simulink model "PubIfDecisionLM_MDL"  (R2020b)
settings: configuration reference "DspaceConfig" (kept outside this file)
PostLoadFcn:
  | if any(exist('dsrtsu_mdlpostloadfcn', 'file') ~= 0), dsrtsu_mdlpostloadfcn('Execute', bdroot); end
InitFcn:
  | , if any(exist('dsmpb_private', 'file') ~= 0), dsmpb_private('dsmpb_mdlclblib', 'Init', bdroot); end,
undefined symbols (not defined in the file or in its folder): OFM_OBJ_FUSIONTYPE_E, OFM_OBJ_MOVINGSTATE_E, OFM_OBJ_ORIENTATION_E, OFM_OBJ_TYPE_E, P_LM_Cyc, P_LM_EMLHistKapRcdBufSize, P_LM_EMLHistTrajBaseDis, P_LM_EMLHistTrajPNum, P_LM_EMLKapCorrMaxThre, P_LM_EMLMinKapThre, P_LM_EMLPathDisDiffThre, P_LM_EMLQuaFiltPar, P_LM_EMLTurnActKapThre, P_LM_EMLValidQuaThre, P_LM_FntPath1Disgap, P_LM_FntPath1MinDis, P_LM_FntPath1Timegap, P_LM_FntPath2Disgap, P_LM_FntPath2MinDis, P_LM_FntPath2Timegap, P_LM_FntPath3Disgap, P_LM_FntPath3MinDis, P_LM_FntPath3Timegap, P_LM_FusBLParFiltP, P_LM_FusEVDifC2Thre, P_LM_FusEVOPath1AllVSLDisThre, P_LM_FusEVOPath1AllVSLLostNumThre, P_LM_FusEVOPath1AllVSLQuaThre, P_LM_FusEVOPath1OTLFacNLC, P_LM_FusOTLQuaThre, P_LM_FusOTLSW, P_LM_FusParC0Index, P_LM_FusParC1Index, P_LM_FusParC2Index, P_LM_FusParC3Index, P_LM_FusVSLQuaThre, P_LM_FusVSLSW, P_LM_FusVSLValidSteerWheerAngThre, P_LM_FusVSLValidVxvThre, P_LM_LaneWidth, P_LM_OTLBufTPInfoEvaFactor, P_LM_OTLObjNum, P_LM_OTLObjSelectAgeThre, P_LM_OTLObjSelectDxAssessVx, P_LM_OTLObjSelectDxThre, P_LM_OTLObjSelectVxThre, P_LM_OTLObjSelectVyAssessDx, P_LM_OTLObjSelectVyThre, P_LM_OTLTrajPntBaseDis, P_LM_OTLTrajStdThre, P_LM_VSLAvailLineNum, P_LM_VSLBLSDiffThre, P_LM_VSLBLSDisRatio, P_LM_VSLFusBLParFiltP_C1, P_LM_VSLFusBLParFiltP_C2, P_LM_VSLFusBLParFiltP_C3, P_LM_VSLFusBLParFiltP_Quality, P_LM_VSLHistTrajBaseDis, P_LM_VSLHistTrajPNum, P_LM_VSLLCC0diff ... (+18)
libraries: simulink x145, LM_LIB x43
(part 3 of 24)

== system PubIfDecisionLM_MDL/Subsystem2/LM_EML/LM_EMLFntPath1/LM_EML_C0 ==
  LM_DrivInWLType : Inport
  Constant : Constant  Value=P_LM_LaneWidth  OutDataTypeStr=single
  Merge{,1..3} (4 alike) : Merge  Inputs=3
  Switch Case : SwitchCase  CaseConditions={[0,2],1,3}  ShowDefaultCase=off
  Switch Case Action Subsystem : Subsystem  TreatAsAtomicUnit=on
  Switch Case Action Subsystem1 : Subsystem  TreatAsAtomicUnit=on
  Switch Case Action Subsystem2 : Subsystem  TreatAsAtomicUnit=on
  LM_EMLLLC0 : Outport
  LM_EMLLRC0 : Outport  Port=2
  LM_EMLRLC0 : Outport  Port=3
  LM_EMLRRC0 : Outport  Port=4
  wires:
  Merge3/1 -> LM_EMLRRC0/1  "LM_EMLRRC0"
  Merge2/1 -> LM_EMLRLC0/1  "LM_EMLRLC0"
  Merge1/1 -> LM_EMLLRC0/1  "LM_EMLLRC0"
  Switch Case Action Subsystem2/4(LM_EML_RRC0) -> Merge3/3
  Switch Case Action Subsystem1/4(LM_EML_RRC0) -> Merge3/2
  Switch Case Action Subsystem/4(LM_EML_RRC0) -> Merge3/1
  Switch Case Action Subsystem2/3(LM_EML_RLC0) -> Merge2/3
  Switch Case Action Subsystem1/3(LM_EML_RLC0) -> Merge2/2
  Switch Case Action Subsystem1/2(LM_EML_LRC0) -> Merge1/2
  Switch Case Action Subsystem1/1(LM_EML_LLC0) -> Merge/2
  Switch Case Action Subsystem/3(LM_EML_RLC0) -> Merge2/1
  Switch Case Action Subsystem2/2(LM_EML_LRC0) -> Merge1/3
  Switch Case Action Subsystem/2(LM_EML_LRC0) -> Merge1/1
  Switch Case Action Subsystem2/1(LM_EML_LLC0) -> Merge/3
  Merge/1 -> LM_EMLLLC0/1  "LM_EMLLLC0"
  Switch Case Action Subsystem/1(LM_EML_LLC0) -> Merge/1
  Constant/1 -> Switch Case Action Subsystem/1(P_LM_LaneWidth), Switch Case Action Subsystem1/1(P_LM_LaneWidth), Switch Case Action Subsystem2/1(P_LM_LaneWidth)
  Switch Case/3 -> Switch Case Action Subsystem2/Action
  Switch Case/2 -> Switch Case Action Subsystem1/Action
  Switch Case/1 -> Switch Case Action Subsystem/Action
  LM_DrivInWLType/1 -> Switch Case/1

== system PubIfDecisionLM_MDL/Subsystem2/LM_EML/LM_EMLRearPath1/LM_EMLEgoTrajRecorddFlgCalc ==
  note: 0x0: not standstill
  VehStandstill : Inport
  VxvRef_ms : Inport  Port=2
  Add : Sum
  Compare To Zero : simulink/Logic and Bit Operations/Compare To Zero  relop===  OutDataTypeStr=boolean
  Constant : Constant  Value=0  OutDataTypeStr=boolean
  Constant1 : Constant  OutDataTypeStr=uint8
  Constant2 : Constant  Value=0
  Constant3 : Constant  Value=0.0001  OutDataTypeStr=single
  Constant4 : Constant  Value=P_LM_EMLHistTrajBaseDis  OutDataTypeStr=single
  Constant6 : Constant  Value=P_LM_Cyc
  Data Type Conversion : DataTypeConversion  OutDataTypeStr=uint8
  Divide : Product  Inputs=*/
  Divide1 : Product  Inputs=*/
  Relational Operator : RelationalOperator  Operator=<=  OutDataTypeStr=boolean  RndMeth=Nearest
  Switch : Switch  Criteria=u2 ~= 0
  Switch1 : Switch  Criteria=u2 ~= 0
  Switch2 : Switch  Criteria=u2 ~= 0
  Unit Delay : UnitDelay  SampleTime=-1  HasFrameUpgradeWarning=on
  LM_EMLHistTrajRcdFlg : Outport
  wires:
  Constant4/1 -> Divide/1
  Switch2/1 -> Divide/2
  Divide/1 -> Divide1/1
  Constant6/1 -> Divide1/2
  Constant/1 -> Switch/1
  Switch/1 -> LM_EMLHistTrajRcdFlg/1  "LM_EMLHistTrajRcdFlg"
  Unit Delay/1 -> Add/2
  Constant1/1 -> Add/1
  Divide1/1 -> Data Type Conversion/1
  Add/1 -> Relational Operator/2, Switch1/3
  Constant2/1 -> Switch1/1
  Switch1/1 -> Unit Delay/1
  Data Type Conversion/1 -> Relational Operator/1
  Relational Operator/1 -> Switch/3, Switch1/2
  VehStandstill/1 -> Switch/2
  VxvRef_ms/1 -> Switch2/3, Compare To Zero/1
  Compare To Zero/1 -> Switch2/2
  Constant3/1 -> Switch2/1

== system PubIfDecisionLM_MDL/Subsystem2/LM_EML/LM_EMLRearPath1/LM_EMLHistTrajCoordinateConvert ==
  note: 0x0: not standstill
  LM_EMLHistTrajVectXK1 : Inport
  LM_EMLHistTrajVectYK1 : Inport  Port=2
  LM_ComEVOffsetX : Inport  Port=3
  LM_ComEVOffsetY : Inport  Port=4
  LM_ComEVOffsetAng : Inport  Port=5
  VehStandstill : Inport  Port=6
  If : If  IfExpression=u1 == 0
  If Action Subsystem : Subsystem  TreatAsAtomicUnit=on
  If Action Subsystem1 : Subsystem  TreatAsAtomicUnit=on
  Merge : Merge
  Merge1 : Merge
  LM_EMLHistTrajVectXK1Adju : Outport
  LM_EMLHistTrajVectYK1Adju : Outport  Port=2
  wires:
  Merge1/1 -> LM_EMLHistTrajVectYK1Adju/1
  Merge/1 -> LM_EMLHistTrajVectXK1Adju/1
  If Action Subsystem1/2(LM_EMLHistTrajVectYK1Adju) -> Merge1/2
  If Action Subsystem/2(LM_EMLHistTrajVectYK1Adju) -> Merge1/1
  If Action Subsystem1/1(LM_EMLHistTrajVectXK1Adju) -> Merge/2
  If Action Subsystem/1(LM_EMLHistTrajVectXK1Adju) -> Merge/1
  LM_ComEVOffsetX/1 -> If Action Subsystem/1(LM_ComEVOffsetX)
  LM_ComEVOffsetY/1 -> If Action Subsystem/2(LM_ComEVOffsetY)
  LM_ComEVOffsetAng/1 -> If Action Subsystem/3(LM_ComEVOffsetAng)
  LM_EMLHistTrajVectXK1/1 -> If Action Subsystem/4(LM_EMLHistTrajVectXK1), If Action Subsystem1/1(LM_EMLHistTrajVectXK1)
  LM_EMLHistTrajVectYK1/1 -> If Action Subsystem/5(LM_EMLHistTrajVectYK1), If Action Subsystem1/2(LM_EMLHistTrajVectYK1)
  If/2 -> If Action Subsystem1/Action
  If/1 -> If Action Subsystem/Action
  VehStandstill/1 -> If/1

== system PubIfDecisionLM_MDL/Subsystem2/LM_EML/LM_EMLRearPath1/LM_EMLHistTrajRecordBufferInfo ==
  LM_EMLHistTrajRcdFlg : Inport
  Add : Sum
  Add1 : Sum
  Add2 : Sum
  Compare To Zero{,1..3} (4 alike) : simulink/Logic and Bit Operations/Compare To Zero  relop===  OutDataTypeStr=boolean
  Constant{,2..4,7..9} (7 alike) : Constant  OutDataTypeStr=uint8
  Constant1 : Constant  Value=P_LM_EMLHistTrajPNum  OutDataTypeStr=uint8
  Constant5 : Constant  Value=P_LM_EMLHistTrajPNum  OutDataTypeStr=uint8
  Constant6 : Constant  Value=3  OutDataTypeStr=uint8
  Mod1 : Math  Operator=mod  SignedPower=on  SaturateOnIntegerOverflow=on
  Product : Product
  Relational Operator : RelationalOperator  Operator=>  OutDataTypeStr=boolean  RndMeth=Nearest
  Relational Operator1 : RelationalOperator  Operator=<=  OutDataTypeStr=boolean  RndMeth=Nearest
  Switch{,1..7} (8 alike) : Switch  Criteria=u2 ~= 0
  Unit Delay : UnitDelay  SampleTime=-1  HasFrameUpgradeWarning=on
  LM_EMLHistPEndPos : Outport
  LM_EMLHistPFristPos : Outport  Port=2
  LM_EMLHistPNum : Outport  Port=3
  wires:
  Switch2/1 -> Switch5/3  "LM_EMLHistPEndPos"
  Compare To Zero/1 -> Switch2/2
  Switch6/1 -> LM_EMLHistPEndPos/1  "LM_EMLHistPEndPos"
  LM_EMLHistTrajRcdFlg/1 -> Switch1/2
  Switch/1 -> LM_EMLHistPFristPos/1  "LM_EMLHistPFristPos"
  Constant3/1 -> Add2/2
  Mod1/1 -> Add1/1, Compare To Zero/1, Switch2/3
  Add2/1 -> Switch4/1
  Add1/1 -> Switch3/3
  Add/1 -> Switch1/1
  Switch1/1 -> Relational Operator1/1, Mod1/1, Switch4/3, Relational Operator/1, Switch5/1
  Relational Operator1/1 -> Switch3/2, Switch5/2
  Constant5/1 -> Product/1
  Product/1 -> Relational Operator/2
  Constant4/1 -> Add1/2
  Relational Operator/1 -> Switch4/2
  Constant1/1 -> Relational Operator1/2, Mod1/2, Add2/1, Switch2/1
  Constant2/1 -> Switch3/1
  Unit Delay/1 -> Switch1/3, Add/1
  Constant6/1 -> Product/2
  Constant/1 -> Add/2
  Switch3/1 -> Switch/3, Compare To Zero1/1
  Compare To Zero1/1 -> Switch/2
  Constant7/1 -> Switch/1
  Constant8/1 -> Switch6/1
  Compare To Zero2/1 -> Switch6/2
  Switch5/1 -> Compare To Zero2/1, Switch6/3
  Switch4/1 -> Switch7/3, Unit Delay/1, Compare To Zero3/1
  Compare To Zero3/1 -> Switch7/2
  Constant9/1 -> Switch7/1
  Switch7/1 -> LM_EMLHistPNum/1  "LM_EMLHistPNum"

== system PubIfDecisionLM_MDL/Subsystem2/LM_EML/LM_EMLRearPath1/LM_EMLHistTrajRecordBufferUpdate ==
  LM_EMLHistTrajVectXK1Adju : Inport
  LM_EMLHistTrajVectYK1Adju : Inport  Port=2
  LM_EMLHistTrajRcdFlg : Inport  Port=3
  LM_EMLHistPEndPos : Inport  Port=4
  Data Type Conversion : DataTypeConversion  OutDataTypeStr=single
  Data Type Conversion1 : DataTypeConversion  OutDataTypeStr=single
  MATLAB Function : MATLAB Function  TreatAsAtomicUnit=on
  MATLAB Function1 : MATLAB Function  TreatAsAtomicUnit=on
  Switch : Switch  Criteria=u2 ~= 0
  Switch2 : Switch  Criteria=u2 ~= 0
  LM_EMLHistTrajVectX : Outport
  LM_EMLHistTrajVectY : Outport  Port=2
  wires:
  MATLAB Function1/1(LM_EMLHistTrajVectX) -> Switch2/1
  MATLAB Function/1(LM_EMLHistTrajVectX) -> Switch/1
  LM_EMLHistPEndPos/1 -> MATLAB Function/1(LM_EMLHistPEndPos), MATLAB Function1/1(LM_EMLHistPEndPos)
  LM_EMLHistTrajVectXK1Adju/1 -> MATLAB Function/2(LM_EMLHistTrajVectXK1Adju), Switch/3
  LM_EMLHistTrajRcdFlg/1 -> Switch2/2, Switch/2
  LM_EMLHistTrajVectYK1Adju/1 -> Switch2/3, MATLAB Function1/2(LM_EMLHistTrajVectXK1Adju)
  Switch2/1 -> Data Type Conversion1/1
  Switch/1 -> Data Type Conversion/1
  Data Type Conversion/1 -> LM_EMLHistTrajVectX/1
  Data Type Conversion1/1 -> LM_EMLHistTrajVectY/1

== system PubIfDecisionLM_MDL/Subsystem2/LM_Fusion1/LM_FusBaseLineFilt/LM_FusBaseLineC0Filt ==
  note: P_LM_FusBLParFiltP
  note: P_LM_FusBLParFiltP
  note: P_LM_FusBLParFiltP
  note: P_LM_FusBLParFiltP
  DIR_LC2LeValid : Inport
  DIR_LC2RigValid : Inport  Port=2
  LM_LLC0BefFilt : Inport  Port=3
  LM_LRC0BefFilt : Inport  Port=4
  LM_RLC0BefFilt : Inport  Port=5
  LM_RRC0BefFilt : Inport  Port=6
  Add{1..3,12} (4 alike) : Sum
  Compare To Zero{,1..3} (4 alike) : simulink/Logic and Bit Operations/Compare To Zero  relop===  OutDataTypeStr=boolean
  Constant{1..3,10} (4 alike) : Constant  Value=P_LM_FusBLParFiltP  OutDataTypeStr=single
  Logical Operator : Logic  Operator=OR  AllPortsSameDT=off  OutDataTypeStr=boolean
  Product{1..3,17} (4 alike) : Product
  Subtract{1..4} (4 alike) : Sum  Inputs=+-
  Switch{,1..7} (8 alike) : Switch  Criteria=u2 ~= 0
  Unit Delay{1..4} (4 alike) : UnitDelay  SampleTime=-1  HasFrameUpgradeWarning=on
  LM_LLC0 : Outport
  LM_LRC0 : Outport  Port=2
  LM_RLC0 : Outport  Port=3
  LM_RRC0 : Outport  Port=4
  wires:
  Constant10/1 -> Product17/2
  Add12/1 -> Switch4/3
  Unit Delay2/1 -> Compare To Zero/1, Add12/2, Subtract2/2
  Subtract2/1 -> Product17/1
  Product17/1 -> Add12/1
  LM_LLC0BefFilt/1 -> Subtract2/1, Switch4/1, Switch/1
  DIR_LC2LeValid/1 -> Logical Operator/1
  DIR_LC2RigValid/1 -> Logical Operator/2
  Logical Operator/1 -> Switch3/2, Switch2/2, Switch1/2, Switch/2
  Constant1/1 -> Product1/2
  Add1/1 -> Switch5/3
  Unit Delay1/1 -> Compare To Zero1/1, Add1/2, Subtract1/2
  Subtract1/1 -> Product1/1
  Product1/1 -> Add1/1
  LM_LRC0BefFilt/1 -> Switch5/1, Switch1/1, Subtract1/1
  Product2/1 -> Add2/1
  Subtract3/1 -> Product2/1
  Unit Delay3/1 -> Compare To Zero2/1, Add2/2, Subtract3/2
  Constant2/1 -> Product2/2
  LM_RLC0BefFilt/1 -> Switch6/1, Switch2/1, Subtract3/1
  Product3/1 -> Add3/1
  Subtract4/1 -> Product3/1
  Unit Delay4/1 -> Compare To Zero3/1, Add3/2, Subtract4/2
  Constant3/1 -> Product3/2
  Switch/1 -> LM_LLC0/1, Unit Delay2/1  "LM_LLC0"
  Switch1/1 -> LM_LRC0/1, Unit Delay1/1  "LM_LRC0"
  Switch2/1 -> LM_RLC0/1, Unit Delay3/1  "LM_RLC0"
  Switch3/1 -> LM_RRC0/1, Unit Delay4/1  "LM_RRC0"
  Switch4/1 -> Switch/3  "LM_LLC0"
  Compare To Zero/1 -> Switch4/2
  Compare To Zero1/1 -> Switch5/2
  Switch5/1 -> Switch1/3  "LM_LLC0"
  Switch6/1 -> Switch2/3  "LM_LLC0"
  Add2/1 -> Switch6/3
  Compare To Zero2/1 -> Switch6/2
  Compare To Zero3/1 -> Switch7/2
  Add3/1 -> Switch7/3
  LM_RRC0BefFilt/1 -> Subtract4/1, Switch3/1, Switch7/1
  Switch7/1 -> Switch3/3  "LM_LLC0"

== system PubIfDecisionLM_MDL/Subsystem2/LM_Fusion1/LM_FusBaseLineFilt/LM_FusBaseLineInfoFilt ==
  LM_FusBLInfo : Inport
  Bus Creator{,1..5} (6 alike) : BusCreator  Inputs=5  OutDataTypeStr=Bus: LM_FusBLPathInfoBus
  Bus Selector : BusSelector  OutputSignals=LM_FusBLFntPath1Info.LM_FusBLPathC0,LM_FusBLFntPath1Info.LM_FusBLPathC1,LM_FusBLFntPath1Info.LM_FusBLPathC2,LM_FusBLFntPath1Info.LM_FusBLPathC3,LM_FusBLFntPath1Info.LM_FusBLPathQuality
  Bus Selector1 : BusSelector  OutputSignals=LM_FusBLFntPath2Info.LM_FusBLPathC0,LM_FusBLFntPath2Info.LM_FusBLPathC1,LM_FusBLFntPath2Info.LM_FusBLPathC2,LM_FusBLFntPath2Info.LM_FusBLPathC3,LM_FusBLFntPath2Info.LM_FusBLPathQuality
  Bus Selector2 : BusSelector  OutputSignals=LM_FusBLFntPath3Info.LM_FusBLPathC0,LM_FusBLFntPath3Info.LM_FusBLPathC1,LM_FusBLFntPath3Info.LM_FusBLPathC2,LM_FusBLFntPath3Info.LM_FusBLPathC3,LM_FusBLFntPath3Info.LM_FusBLPathQuality
  Bus Selector3 : BusSelector  OutputSignals=LM_FusBLRearPath1Info.LM_FusBLPathC0,LM_FusBLRearPath1Info.LM_FusBLPathC1,LM_FusBLRearPath1Info.LM_FusBLPathC2,LM_FusBLRearPath1Info.LM_FusBLPathC3,LM_FusBLRearPath1Info.LM_FusBLPathQuality
  Bus Selector4 : BusSelector  OutputSignals=LM_FusBLRearPath2Info.LM_FusBLPathC0,LM_FusBLRearPath2Info.LM_FusBLPathC1,LM_FusBLRearPath2Info.LM_FusBLPathC2,LM_FusBLRearPath2Info.LM_FusBLPathC3,LM_FusBLRearPath2Info.LM_FusBLPathQuality
  Bus Selector5 : BusSelector  OutputSignals=LM_FusBLRearPath3Info.LM_FusBLPathC0,LM_FusBLRearPath3Info.LM_FusBLPathC1,LM_FusBLRearPath3Info.LM_FusBLPathC2,LM_FusBLRearPath3Info.LM_FusBLPathC3,LM_FusBLRearPath3Info.LM_FusBLPathQuality
  LM_FusBLFntPath1InfoFilt : Subsystem
  LM_FusBLFntPath2InfoFilt : LM_LIB/LM_FusBLPathInfoFilt  SystemSampleTime=-1  VariantActivationTime=update diagram  Latency=0  AutoFrameSizeCalculation=off
  LM_FusBLFntPath3InfoFilt : LM_LIB/LM_FusBLPathInfoFilt  SystemSampleTime=-1  VariantActivationTime=update diagram  Latency=0  AutoFrameSizeCalculation=off
  LM_FusBLRearPath1InfoFilt : LM_LIB/LM_FusBLPathInfoFilt  SystemSampleTime=-1  VariantActivationTime=update diagram  Latency=0  AutoFrameSizeCalculation=off
  LM_FusBLRearPath2InfoFilt : LM_LIB/LM_FusBLPathInfoFilt  SystemSampleTime=-1  VariantActivationTime=update diagram  Latency=0  AutoFrameSizeCalculation=off
  LM_FusBLRearPath3InfoFilt : LM_LIB/LM_FusBLPathInfoFilt  SystemSampleTime=-1  VariantActivationTime=update diagram  Latency=0  AutoFrameSizeCalculation=off
  Signal Conversion{,1..29} (30 alike) : SignalConversion  OverrideOpt=off
  LM_FusBLFntPath1Info : Outport
  LM_FusBLFntPath2Info : Outport  Port=2
  LM_FusBLFntPath3Info : Outport  Port=3
  LM_FusBLRearPath1Info : Outport  Port=4
  LM_FusBLRearPath2Info : Outport  Port=5
  LM_FusBLRearPath3Info : Outport  Port=6
  wires:
  Bus Selector/1 -> LM_FusBLFntPath1InfoFilt/1(LM_FusBLPathC0)  "<LM_FusBLPathC0>"
  Bus Selector/2 -> LM_FusBLFntPath1InfoFilt/2(LM_FusBLPathC1)  "<LM_FusBLPathC1>"
  Bus Selector/3 -> LM_FusBLFntPath1InfoFilt/3(LM_FusBLPathC2)  "<LM_FusBLPathC2>"
  Bus Selector/4 -> LM_FusBLFntPath1InfoFilt/4(LM_FusBLPathC3)  "<LM_FusBLPathC3>"
  Bus Selector/5 -> LM_FusBLFntPath1InfoFilt/5(LM_FusBLPathQuality)  "<LM_FusBLPathQuality>"
  Bus Creator/1 -> LM_FusBLFntPath1Info/1  "LM_FusBLFntPath1Info"
  LM_FusBLFntPath1InfoFilt/1(LM_FusBLPathC0Filt) -> Signal Conversion/1
  LM_FusBLFntPath1InfoFilt/2(LM_FusBLPathC1Filt) -> Signal Conversion1/1
  LM_FusBLFntPath1InfoFilt/3(LM_FusBLPathC2Filt) -> Signal Conversion2/1
  LM_FusBLFntPath1InfoFilt/4(LM_FusBLPathC3Filt) -> Signal Conversion3/1
  LM_FusBLFntPath1InfoFilt/5(LM_FusBLPathQualityFilt) -> Signal Conversion4/1
  LM_FusBLFntPath2InfoFilt/5 -> Signal Conversion9/1
  LM_FusBLFntPath2InfoFilt/4 -> Signal Conversion8/1
  LM_FusBLFntPath2InfoFilt/3 -> Signal Conversion7/1
  LM_FusBLFntPath2InfoFilt/2 -> Signal Conversion6/1
  LM_FusBLFntPath2InfoFilt/1 -> Signal Conversion5/1
  Bus Creator1/1 -> LM_FusBLFntPath2Info/1  "LM_FusBLFntPath2Info"
  Bus Creator2/1 -> LM_FusBLFntPath3Info/1  "LM_FusBLFntPath3Info"
  LM_FusBLFntPath3InfoFilt/1 -> Signal Conversion10/1
  LM_FusBLFntPath3InfoFilt/2 -> Signal Conversion11/1
  LM_FusBLFntPath3InfoFilt/3 -> Signal Conversion12/1
  LM_FusBLFntPath3InfoFilt/4 -> Signal Conversion13/1
  LM_FusBLFntPath3InfoFilt/5 -> Signal Conversion14/1
  LM_FusBLRearPath1InfoFilt/5 -> Signal Conversion24/1
  LM_FusBLRearPath1InfoFilt/4 -> Signal Conversion23/1
  LM_FusBLRearPath1InfoFilt/3 -> Signal Conversion22/1
  LM_FusBLRearPath1InfoFilt/2 -> Signal Conversion16/1
  LM_FusBLRearPath1InfoFilt/1 -> Signal Conversion15/1
  Bus Creator3/1 -> LM_FusBLRearPath1Info/1  "LM_FusBLRearPath1Info"
  Bus Creator4/1 -> LM_FusBLRearPath2Info/1  "LM_FusBLRearPath2Info"
  LM_FusBLRearPath2InfoFilt/1 -> Signal Conversion17/1
  LM_FusBLRearPath2InfoFilt/2 -> Signal Conversion18/1
  LM_FusBLRearPath2InfoFilt/3 -> Signal Conversion19/1
  LM_FusBLRearPath2InfoFilt/4 -> Signal Conversion20/1
  LM_FusBLRearPath2InfoFilt/5 -> Signal Conversion21/1
  LM_FusBLRearPath3InfoFilt/5 -> Signal Conversion29/1
  LM_FusBLRearPath3InfoFilt/4 -> Signal Conversion28/1
  LM_FusBLRearPath3InfoFilt/3 -> Signal Conversion27/1
  LM_FusBLRearPath3InfoFilt/2 -> Signal Conversion26/1
  LM_FusBLRearPath3InfoFilt/1 -> Signal Conversion25/1
  Bus Creator5/1 -> LM_FusBLRearPath3Info/1  "LM_FusBLRearPath3Info"
  Bus Selector1/1 -> LM_FusBLFntPath2InfoFilt/1  "<LM_FusBLPathC0>"
  Bus Selector1/2 -> LM_FusBLFntPath2InfoFilt/2  "<LM_FusBLPathC1>"
  Bus Selector1/3 -> LM_FusBLFntPath2InfoFilt/3  "<LM_FusBLPathC2>"
  Bus Selector1/4 -> LM_FusBLFntPath2InfoFilt/4  "<LM_FusBLPathC3>"
  Bus Selector1/5 -> LM_FusBLFntPath2InfoFilt/5  "<LM_FusBLPathQuality>"
  Bus Selector2/1 -> LM_FusBLFntPath3InfoFilt/1  "<LM_FusBLPathC0>"
  Bus Selector2/2 -> LM_FusBLFntPath3InfoFilt/2  "<LM_FusBLPathC1>"
  Bus Selector2/3 -> LM_FusBLFntPath3InfoFilt/3  "<LM_FusBLPathC2>"
  Bus Selector2/4 -> LM_FusBLFntPath3InfoFilt/4  "<LM_FusBLPathC3>"
  Bus Selector2/5 -> LM_FusBLFntPath3InfoFilt/5  "<LM_FusBLPathQuality>"
  Bus Selector5/5 -> LM_FusBLRearPath3InfoFilt/5  "<LM_FusBLPathQuality>"
  Bus Selector5/4 -> LM_FusBLRearPath3InfoFilt/4  "<LM_FusBLPathC3>"
  Bus Selector5/3 -> LM_FusBLRearPath3InfoFilt/3  "<LM_FusBLPathC2>"
  Bus Selector5/2 -> LM_FusBLRearPath3InfoFilt/2  "<LM_FusBLPathC1>"
  Bus Selector5/1 -> LM_FusBLRearPath3InfoFilt/1  "<LM_FusBLPathC0>"
  LM_FusBLInfo/1 -> Bus Selector3/1, Bus Selector4/1, Bus Selector5/1, Bus Selector2/1, Bus Selector1/1, Bus Selector/1
  Bus Selector4/5 -> LM_FusBLRearPath2InfoFilt/5  "<LM_FusBLPathQuality>"
  Bus Selector4/4 -> LM_FusBLRearPath2InfoFilt/4  "<LM_FusBLPathC3>"
  Bus Selector4/3 -> LM_FusBLRearPath2InfoFilt/3  "<LM_FusBLPathC2>"
  Bus Selector4/2 -> LM_FusBLRearPath2InfoFilt/2  "<LM_FusBLPathC1>"
  Bus Selector4/1 -> LM_FusBLRearPath2InfoFilt/1  "<LM_FusBLPathC0>"
  Bus Selector3/5 -> LM_FusBLRearPath1InfoFilt/5  "<LM_FusBLPathQuality>"
  Bus Selector3/4 -> LM_FusBLRearPath1InfoFilt/4  "<LM_FusBLPathC3>"
  Bus Selector3/3 -> LM_FusBLRearPath1InfoFilt/3  "<LM_FusBLPathC2>"
  Bus Selector3/2 -> LM_FusBLRearPath1InfoFilt/2  "<LM_FusBLPathC1>"
  Bus Selector3/1 -> LM_FusBLRearPath1InfoFilt/1  "<LM_FusBLPathC0>"
  Signal Conversion4/1 -> Bus Creator/5  "LM_FusBLPathQuality"
  Signal Conversion3/1 -> Bus Creator/4  "LM_FusBLPathC3"
  Signal Conversion2/1 -> Bus Creator/3  "LM_FusBLPathC2"
  Signal Conversion1/1 -> Bus Creator/2  "LM_FusBLPathC1"
  Signal Conversion/1 -> Bus Creator/1  "LM_FusBLPathC0"
  Signal Conversion5/1 -> Bus Creator1/1  "LM_FusBLPathC0"
  Signal Conversion6/1 -> Bus Creator1/2  "LM_FusBLPathC1"
  Signal Conversion7/1 -> Bus Creator1/3  "LM_FusBLPathC2"
  Signal Conversion8/1 -> Bus Creator1/4  "LM_FusBLPathC3"
  Signal Conversion9/1 -> Bus Creator1/5  "LM_FusBLPathQuality"
  Signal Conversion24/1 -> Bus Creator3/5  "LM_FusBLPathQuality"
  Signal Conversion23/1 -> Bus Creator3/4  "LM_FusBLPathC3"
  Signal Conversion22/1 -> Bus Creator3/3  "LM_FusBLPathC2"
  Signal Conversion16/1 -> Bus Creator3/2  "LM_FusBLPathC1"
  Signal Conversion15/1 -> Bus Creator3/1  "LM_FusBLPathC0"
  Signal Conversion10/1 -> Bus Creator2/1  "LM_FusBLPathC0"
  Signal Conversion11/1 -> Bus Creator2/2  "LM_FusBLPathC1"
  Signal Conversion12/1 -> Bus Creator2/3  "LM_FusBLPathC2"
  Signal Conversion13/1 -> Bus Creator2/4  "LM_FusBLPathC3"
  Signal Conversion14/1 -> Bus Creator2/5  "LM_FusBLPathQuality"
  Signal Conversion21/1 -> Bus Creator4/5  "LM_FusBLPathQuality"
  Signal Conversion20/1 -> Bus Creator4/4  "LM_FusBLPathC3"
  Signal Conversion19/1 -> Bus Creator4/3  "LM_FusBLPathC2"
  Signal Conversion18/1 -> Bus Creator4/2  "LM_FusBLPathC1"
  Signal Conversion17/1 -> Bus Creator4/1  "LM_FusBLPathC0"
  Signal Conversion25/1 -> Bus Creator5/1  "LM_FusBLPathC0"
  Signal Conversion26/1 -> Bus Creator5/2  "LM_FusBLPathC1"
  Signal Conversion27/1 -> Bus Creator5/3  "LM_FusBLPathC2"
  Signal Conversion28/1 -> Bus Creator5/4  "LM_FusBLPathC3"
  Signal Conversion29/1 -> Bus Creator5/5  "LM_FusBLPathQuality"

== system PubIfDecisionLM_MDL/Subsystem2/LM_Fusion1/LM_FusBaseLineFilt/Subsystem1 ==
  Bus Creator : BusCreator  Inputs=5
  Bus Creator1 : BusCreator  Inputs=5
  Bus Creator2 : BusCreator  Inputs=5
  LM_FusBLFntPath1Info : Outport
  LM_FusBLFntPath2Info : Outport  Port=2
  LM_FusBLFntPath3Info : Outport  Port=3
  wires:
  ? -> Bus Creator/1  "LM_FusBLFntPath1C0"
  Bus Creator/1 -> LM_FusBLFntPath1Info/1  "LM_FusBLFntPath1Info"
  Bus Creator2/1 -> LM_FusBLFntPath3Info/1  "LM_FusBLFntPath3Info"
  ? -> Bus Creator1/4  "LM_FusBLFntPath2C3"
  ? -> Bus Creator/3  "LM_FusBLFntPath1C2"
  ? -> Bus Creator2/2  "LM_FusBLFntPath3C1"
  ? -> Bus Creator/4  "LM_FusBLFntPath1C3"
  ? -> Bus Creator2/3  "LM_FusBLFntPath3C2"
  ? -> Bus Creator2/5  "LM_FusBLFntPath3Quality"
  ? -> Bus Creator1/1  "LM_FusBLFntPath2C0"
  ? -> Bus Creator1/2  "LM_FusBLFntPath2C1"
  ? -> Bus Creator2/4  "LM_FusBLFntPath3C3"
  Bus Creator1/1 -> LM_FusBLFntPath2Info/1  "LM_FusBLFntPath2Info"
  ? -> Bus Creator/5  "LM_FusBLFntPath1Quality"
  ? -> Bus Creator2/1  "LM_FusBLFntPath3C0"
  ? -> Bus Creator1/3  "LM_FusBLFntPath2C2"
  ? -> Bus Creator/2  "LM_FusBLFntPath1C1"
  ? -> Bus Creator1/5  "LM_FusBLFntPath2Quality"

== system PubIfDecisionLM_MDL/Subsystem2/LM_Fusion1/LM_FusBaseLineInfoCalc/LM_FusBLFntPath1 ==
  LM_EML : Inport
  LM_VSL : Inport  Port=2
  LM_OTL : Inport  Port=3
  LM_REL : Inport  Port=4
  LM_MAL : Inport  Port=5
  LM_FusFntPathK : Inport  Port=6
  Bus Creator : BusCreator  Inputs=5
  Bus Creator1 : BusCreator  Inputs=5
  Bus Creator2 : BusCreator  Inputs=5
  Bus Selector : BusSelector  OutputSignals=LM_VSLFntPath1P,LM_VSLFntPath1Quality
  Bus Selector1 : BusSelector  OutputSignals=LM_EMLFntPath1P,LM_EMLFntPath1Quality
  Bus Selector10 : BusSelector  OutputSignals=LM_OTLFntPath2P,LM_OTLFntPath2Qulity
  Bus Selector11 : BusSelector  OutputSignals=LM_OTLFntPath3P,LM_OTLFntPath3Qulity
  Bus Selector2 : BusSelector  OutputSignals=LM_FusFntPath1EMLK,LM_FusFntPath1VSLK,LM_FusFntPath1OTLK
  Bus Selector3 : BusSelector  OutputSignals=LM_VSLFntPath2P,LM_VSLFntPath2Quality
  Bus Selector4 : BusSelector  OutputSignals=LM_EMLFntPath2P,LM_EMLFntPath2Quality
  Bus Selector5 : BusSelector  OutputSignals=LM_FusFntPath2EMLK,LM_FusFntPath2VSLK,LM_FusFntPath2OTLK
  Bus Selector6 : BusSelector  OutputSignals=LM_VSLFntPath3P,LM_VSLFntPath3Quality
  Bus Selector7 : BusSelector  OutputSignals=LM_EMLFntPath3P,LM_EMLFntPath3Quality
  Bus Selector8 : BusSelector  OutputSignals=LM_FusFntPath3EMLK,LM_FusFntPath3VSLK,LM_FusFntPath3OTLK
  Bus Selector9 : BusSelector  OutputSignals=LM_OTLFntPath1P,LM_OTLFntPath1Qulity
  Display : Display
  Display1 : Display
  Display2 : Display
  LM_EVOFFntPath1 : Subsystem
  LM_EVOFFntPath2 : Subsystem
  LM_EVOFFntPath3 : Subsystem
  LM_FusBLFntPath1Info : Outport
  LM_FusBLFntPath2Info : Outport  Port=2
  LM_FusBLFntPath3Info : Outport  Port=3
  wires:
  Bus Selector5/2 -> LM_EVOFFntPath2/8(LM_FusFntPath2VSLK)  "<LM_FusFntPath2VSLK>"
  Bus Selector2/1 -> LM_EVOFFntPath1/7(LM_FusFntPath1EMLK)  "<LM_FusFntPath1EMLK>"
  LM_EVOFFntPath3/5(LM_FusBLFntPath3Quality) -> Bus Creator2/5
  LM_EVOFFntPath3/4(LM_FusBLFntPath3C3) -> Bus Creator2/4
  LM_EVOFFntPath3/3(LM_FusBLFntPath3C2) -> Bus Creator2/3
  LM_EVOFFntPath3/2(LM_FusBLFntPath3C1) -> Bus Creator2/2
  LM_EVOFFntPath3/1(LM_FusBLFntPath3C0) -> Bus Creator2/1
  Bus Selector8/3 -> LM_EVOFFntPath3/9(LM_FusFntPath3OTLK)  "<LM_FusFntPath3OTLK>"
  Bus Selector11/2 -> LM_EVOFFntPath3/6(LM_OTLFntPath3Quality)  "<LM_OTLFntPath3Qulity>"
  Bus Selector11/1 -> LM_EVOFFntPath3/5(LM_OTLFntPath3P)  "<LM_OTLFntPath3P>"
  LM_EVOFFntPath2/5(LM_FusBLFntPath2Quality) -> Bus Creator1/5
  LM_EVOFFntPath2/4(LM_FusBLFntPath2C3) -> Bus Creator1/4
  LM_EVOFFntPath2/3(LM_FusBLFntPath2C2) -> Bus Creator1/3
  LM_EVOFFntPath2/2(LM_FusBLFntPath2C1) -> Bus Creator1/2
  LM_EVOFFntPath2/1(LM_FusBLFntPath2C0) -> Bus Creator1/1
  Bus Selector5/3 -> LM_EVOFFntPath2/9(LM_FusFntPath2OTLK)  "<LM_FusFntPath2OTLK>"
  Bus Selector10/2 -> LM_EVOFFntPath2/6(LM_OTLFntPath2Quality)  "<LM_OTLFntPath2Qulity>"
  Bus Selector10/1 -> LM_EVOFFntPath2/5(LM_OTLFntPath2P)  "<LM_OTLFntPath2P>"
  Bus Selector2/3 -> LM_EVOFFntPath1/9(LM_FusFntPath1OTLK)  "<LM_FusFntPath1OTLK>"
  LM_OTL/1 -> Bus Selector9/1, Bus Selector10/1, Bus Selector11/1
  Bus Selector9/2 -> LM_EVOFFntPath1/6(LM_OTLFntPath1Quality)  "<LM_OTLFntPath1Qulity>"
  Bus Selector9/1 -> LM_EVOFFntPath1/5(LM_OTLFntPath1P)  "<LM_OTLFntPath1P>"
  LM_EVOFFntPath1/5(LM_FusBLFntPath1Quality) -> Bus Creator/5
  LM_EVOFFntPath1/4(LM_FusBLFntPath1C3) -> Bus Creator/4
  LM_EVOFFntPath1/3(LM_FusBLFntPath1C2) -> Bus Creator/3
  LM_EVOFFntPath1/2(LM_FusBLFntPath1C1) -> Bus Creator/2
  LM_EVOFFntPath1/1(LM_FusBLFntPath1C0) -> Bus Creator/1
  Bus Selector8/2 -> LM_EVOFFntPath3/8(LM_FusFntPath3VSLK)  "<LM_FusFntPath3VSLK>"
  Bus Selector8/1 -> LM_EVOFFntPath3/7(LM_FusFntPath3EMLK)  "<LM_FusFntPath3EMLK>"
  Bus Selector7/2 -> LM_EVOFFntPath3/4(LM_EMLFntPath3Quality)  "<LM_EMLFntPath3Quality>"
  Bus Selector7/1 -> LM_EVOFFntPath3/3(LM_EMLFntPath3P)  "<LM_EMLFntPath3P>"
  Bus Selector6/2 -> LM_EVOFFntPath3/2(LM_VSLFntPath3Quality)  "<LM_VSLFntPath3Quality>"
  Bus Selector6/1 -> LM_EVOFFntPath3/1(LM_VSLFntPath3P)  "<LM_VSLFntPath3P>"
  Bus Selector5/1 -> LM_EVOFFntPath2/7(LM_FusFntPath2EMLK)  "<LM_FusFntPath2EMLK>"
  Bus Selector4/2 -> LM_EVOFFntPath2/4(LM_EMLFntPath2Quality)  "<LM_EMLFntPath2Quality>"
  Bus Selector4/1 -> LM_EVOFFntPath2/3(LM_EMLFntPath2P)  "<LM_EMLFntPath2P>"
  Bus Selector3/2 -> LM_EVOFFntPath2/2(LM_VSLFntPath2Quality)  "<LM_VSLFntPath2Quality>"
  Bus Selector3/1 -> LM_EVOFFntPath2/1(LM_VSLFntPath2P)  "<LM_VSLFntPath2P>"
  Bus Selector1/2 -> LM_EVOFFntPath1/4(LM_EMLFntPath1Quality)  "<LM_EMLFntPath1Quality>"
  Bus Selector/2 -> LM_EVOFFntPath1/2(LM_VSLFntPath1Quality)  "<LM_VSLFntPath1Quality>"
  LM_FusFntPathK/1 -> Bus Selector8/1, Bus Selector5/1, Bus Selector2/1
  LM_VSL/1 -> Bus Selector/1, Bus Selector3/1, Bus Selector6/1
  LM_EML/1 -> Bus Selector1/1, Bus Selector4/1, Bus Selector7/1
  Bus Creator/1 -> LM_FusBLFntPath1Info/1, Display/1  "LM_FusBLFntPath1Info"
  Bus Creator1/1 -> LM_FusBLFntPath2Info/1, Display1/1  "LM_FusBLFntPath2Info"
  Bus Selector1/1 -> LM_EVOFFntPath1/3(LM_EMLFntPath1P)  "<LM_EMLFntPath1P>"
  Bus Creator2/1 -> LM_FusBLFntPath3Info/1, Display2/1  "LM_FusBLFntPath3Info"
  Bus Selector/1 -> LM_EVOFFntPath1/1(LM_VSLFntPath1P)  "<LM_VSLFntPath1P>"
  Bus Selector2/2 -> LM_EVOFFntPath1/8(LM_FusFntPath1VSLK)  "<LM_FusFntPath1VSLK>"

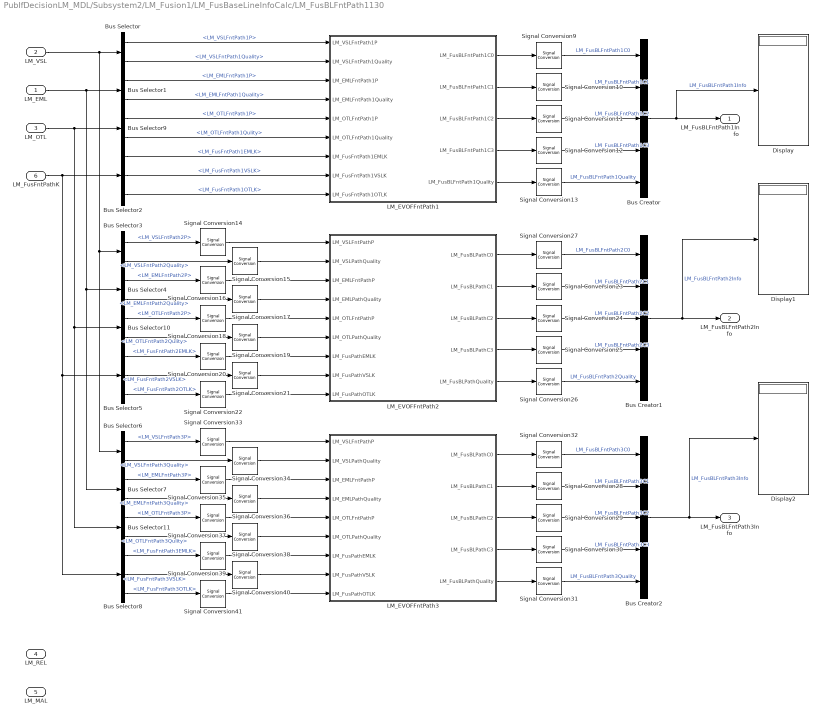
== system PubIfDecisionLM_MDL/Subsystem2/LM_Fusion1/LM_FusBaseLineInfoCalc/LM_FusBLFntPath1130 ==
  LM_EML : Inport
  LM_VSL : Inport  Port=2
  LM_OTL : Inport  Port=3
  LM_REL : Inport  Port=4
  LM_MAL : Inport  Port=5
  LM_FusFntPathK : Inport  Port=6
  Bus Creator : BusCreator  Inputs=5
  Bus Creator1 : BusCreator  Inputs=5
  Bus Creator2 : BusCreator  Inputs=5
  Bus Selector : BusSelector  OutputSignals=LM_VSLFntPath1P,LM_VSLFntPath1Quality
  Bus Selector1 : BusSelector  OutputSignals=LM_EMLFntPath1P,LM_EMLFntPath1Quality
  Bus Selector10 : BusSelector  OutputSignals=LM_OTLFntPath2P,LM_OTLFntPath2Qulity
  Bus Selector11 : BusSelector  OutputSignals=LM_OTLFntPath3P,LM_OTLFntPath3Qulity
  Bus Selector2 : BusSelector  OutputSignals=LM_FusFntPath1EMLK,LM_FusFntPath1VSLK,LM_FusFntPath1OTLK
  Bus Selector3 : BusSelector  OutputSignals=LM_VSLFntPath2P,LM_VSLFntPath2Quality
  Bus Selector4 : BusSelector  OutputSignals=LM_EMLFntPath2P,LM_EMLFntPath2Quality
  Bus Selector5 : BusSelector  OutputSignals=LM_FusFntPath2EMLK,LM_FusFntPath2VSLK,LM_FusFntPath2OTLK
  Bus Selector6 : BusSelector  OutputSignals=LM_VSLFntPath3P,LM_VSLFntPath3Quality
  Bus Selector7 : BusSelector  OutputSignals=LM_EMLFntPath3P,LM_EMLFntPath3Quality
  Bus Selector8 : BusSelector  OutputSignals=LM_FusFntPath3EMLK,LM_FusFntPath3VSLK,LM_FusFntPath3OTLK
  Bus Selector9 : BusSelector  OutputSignals=LM_OTLFntPath1P,LM_OTLFntPath1Qulity
  Display : Display
  Display1 : Display
  Display2 : Display
  LM_EVOFFntPath1 : Subsystem
  LM_EVOFFntPath2 : Subsystem  AncestorBlock=LM_LIB/LM_EVOFusPath
  LM_EVOFFntPath3 : Subsystem  AncestorBlock=LM_LIB/LM_EVOFusPath
  Signal Conversion{9..41} (33 alike) : SignalConversion  OverrideOpt=off
  LM_FusBLFntPath1Info : Outport
  LM_FusBLFntPath2Info : Outport  Port=2
  LM_FusBLFntPath3Info : Outport  Port=3
  wires:
  Signal Conversion41/1 -> LM_EVOFFntPath3/9(LM_FusPathOTLK)
  Signal Conversion40/1 -> LM_EVOFFntPath3/8(LM_FusPathVSLK)
  Signal Conversion39/1 -> LM_EVOFFntPath3/7(LM_FusPathEMLK)
  Signal Conversion38/1 -> LM_EVOFFntPath3/6(LM_OTLPathQuality)
  Signal Conversion37/1 -> LM_EVOFFntPath3/5(LM_OTLFntPathP)
  Signal Conversion36/1 -> LM_EVOFFntPath3/4(LM_EMLPathQuality)
  Signal Conversion34/1 -> LM_EVOFFntPath3/2(LM_VSLPathQuality)
  Signal Conversion35/1 -> LM_EVOFFntPath3/3(LM_EMLFntPathP)
  Signal Conversion33/1 -> LM_EVOFFntPath3/1(LM_VSLFntPathP)
  Signal Conversion20/1 -> LM_EVOFFntPath2/7(LM_FusPathEMLK)
  Signal Conversion18/1 -> LM_EVOFFntPath2/5(LM_OTLFntPathP)
  Signal Conversion21/1 -> LM_EVOFFntPath2/8(LM_FusPathVSLK)
  Signal Conversion15/1 -> LM_EVOFFntPath2/2(LM_VSLPathQuality)
  Signal Conversion19/1 -> LM_EVOFFntPath2/6(LM_OTLPathQuality)
  Signal Conversion17/1 -> LM_EVOFFntPath2/4(LM_EMLPathQuality)
  Signal Conversion16/1 -> LM_EVOFFntPath2/3(LM_EMLFntPathP)
  Signal Conversion14/1 -> LM_EVOFFntPath2/1(LM_VSLFntPathP)
  Signal Conversion22/1 -> LM_EVOFFntPath2/9(LM_FusPathOTLK)
  Signal Conversion32/1 -> Bus Creator2/1  "LM_FusBLFntPath3C0"
  Signal Conversion31/1 -> Bus Creator2/5  "LM_FusBLFntPath3Quality"
  Signal Conversion30/1 -> Bus Creator2/4  "LM_FusBLFntPath3C3"
  Signal Conversion28/1 -> Bus Creator2/2  "LM_FusBLFntPath3C1"
  Signal Conversion29/1 -> Bus Creator2/3  "LM_FusBLFntPath3C2"
  Signal Conversion23/1 -> Bus Creator1/2  "LM_FusBLFntPath2C1"
  Signal Conversion27/1 -> Bus Creator1/1  "LM_FusBLFntPath2C0"
  Signal Conversion26/1 -> Bus Creator1/5  "LM_FusBLFntPath2Quality"
  Signal Conversion25/1 -> Bus Creator1/4  "LM_FusBLFntPath2C3"
  Signal Conversion24/1 -> Bus Creator1/3  "LM_FusBLFntPath2C2"
  Signal Conversion13/1 -> Bus Creator/5  "LM_FusBLFntPath1Quality"
  Signal Conversion12/1 -> Bus Creator/4  "LM_FusBLFntPath1C3"
  Signal Conversion11/1 -> Bus Creator/3  "LM_FusBLFntPath1C2"
  Signal Conversion10/1 -> Bus Creator/2  "LM_FusBLFntPath1C1"
  Signal Conversion9/1 -> Bus Creator/1  "LM_FusBLFntPath1C0"
  Bus Selector5/2 -> Signal Conversion21/1  "<LM_FusFntPath2VSLK>"
  Bus Selector2/1 -> LM_EVOFFntPath1/7(LM_FusFntPath1EMLK)  "<LM_FusFntPath1EMLK>"
  LM_EVOFFntPath3/5(LM_FusBLPathQuality) -> Signal Conversion31/1
  LM_EVOFFntPath3/4(LM_FusBLPathC3) -> Signal Conversion30/1
  LM_EVOFFntPath3/3(LM_FusBLPathC2) -> Signal Conversion29/1
  LM_EVOFFntPath3/2(LM_FusBLPathC1) -> Signal Conversion28/1
  LM_EVOFFntPath3/1(LM_FusBLPathC0) -> Signal Conversion32/1
  Bus Selector8/3 -> Signal Conversion41/1  "<LM_FusFntPath3OTLK>"
  Bus Selector11/2 -> Signal Conversion38/1  "<LM_OTLFntPath3Qulity>"
  Bus Selector11/1 -> Signal Conversion37/1  "<LM_OTLFntPath3P>"
  LM_EVOFFntPath2/5(LM_FusBLPathQuality) -> Signal Conversion26/1
  LM_EVOFFntPath2/4(LM_FusBLPathC3) -> Signal Conversion25/1
  LM_EVOFFntPath2/3(LM_FusBLPathC2) -> Signal Conversion24/1
  LM_EVOFFntPath2/2(LM_FusBLPathC1) -> Signal Conversion23/1
  LM_EVOFFntPath2/1(LM_FusBLPathC0) -> Signal Conversion27/1
  Bus Selector5/3 -> Signal Conversion22/1  "<LM_FusFntPath2OTLK>"
  Bus Selector10/2 -> Signal Conversion19/1  "<LM_OTLFntPath2Qulity>"
  Bus Selector10/1 -> Signal Conversion18/1  "<LM_OTLFntPath2P>"
  Bus Selector2/3 -> LM_EVOFFntPath1/9(LM_FusFntPath1OTLK)  "<LM_FusFntPath1OTLK>"
  LM_OTL/1 -> Bus Selector9/1, Bus Selector10/1, Bus Selector11/1
  Bus Selector9/2 -> LM_EVOFFntPath1/6(LM_OTLFntPath1Quality)  "<LM_OTLFntPath1Qulity>"
  Bus Selector9/1 -> LM_EVOFFntPath1/5(LM_OTLFntPath1P)  "<LM_OTLFntPath1P>"
  LM_EVOFFntPath1/5(LM_FusBLFntPath1Quality) -> Signal Conversion13/1
  LM_EVOFFntPath1/4(LM_FusBLFntPath1C3) -> Signal Conversion12/1
  LM_EVOFFntPath1/3(LM_FusBLFntPath1C2) -> Signal Conversion11/1
  LM_EVOFFntPath1/2(LM_FusBLFntPath1C1) -> Signal Conversion10/1
  LM_EVOFFntPath1/1(LM_FusBLFntPath1C0) -> Signal Conversion9/1
  Bus Selector8/2 -> Signal Conversion40/1  "<LM_FusFntPath3VSLK>"
  Bus Selector8/1 -> Signal Conversion39/1  "<LM_FusFntPath3EMLK>"
  Bus Selector7/2 -> Signal Conversion36/1  "<LM_EMLFntPath3Quality>"
  Bus Selector7/1 -> Signal Conversion35/1  "<LM_EMLFntPath3P>"
  Bus Selector6/2 -> Signal Conversion34/1  "<LM_VSLFntPath3Quality>"
  Bus Selector6/1 -> Signal Conversion33/1  "<LM_VSLFntPath3P>"
  Bus Selector5/1 -> Signal Conversion20/1  "<LM_FusFntPath2EMLK>"
  Bus Selector4/2 -> Signal Conversion17/1  "<LM_EMLFntPath2Quality>"
  Bus Selector4/1 -> Signal Conversion16/1  "<LM_EMLFntPath2P>"
  Bus Selector3/2 -> Signal Conversion15/1  "<LM_VSLFntPath2Quality>"
  Bus Selector3/1 -> Signal Conversion14/1  "<LM_VSLFntPath2P>"
  Bus Selector1/2 -> LM_EVOFFntPath1/4(LM_EMLFntPath1Quality)  "<LM_EMLFntPath1Quality>"
  Bus Selector/2 -> LM_EVOFFntPath1/2(LM_VSLFntPath1Quality)  "<LM_VSLFntPath1Quality>"
  LM_FusFntPathK/1 -> Bus Selector8/1, Bus Selector5/1, Bus Selector2/1
  LM_VSL/1 -> Bus Selector/1, Bus Selector3/1, Bus Selector6/1
  LM_EML/1 -> Bus Selector1/1, Bus Selector4/1, Bus Selector7/1
  Bus Creator/1 -> LM_FusBLFntPath1Info/1, Display/1  "LM_FusBLFntPath1Info"
  Bus Creator1/1 -> LM_FusBLFntPath2Info/1, Display1/1  "LM_FusBLFntPath2Info"
  Bus Selector1/1 -> LM_EVOFFntPath1/3(LM_EMLFntPath1P)  "<LM_EMLFntPath1P>"
  Bus Creator2/1 -> LM_FusBLFntPath3Info/1, Display2/1  "LM_FusBLFntPath3Info"
  Bus Selector/1 -> LM_EVOFFntPath1/1(LM_VSLFntPath1P)  "<LM_VSLFntPath1P>"
  Bus Selector2/2 -> LM_EVOFFntPath1/8(LM_FusFntPath1VSLK)  "<LM_FusFntPath1VSLK>"

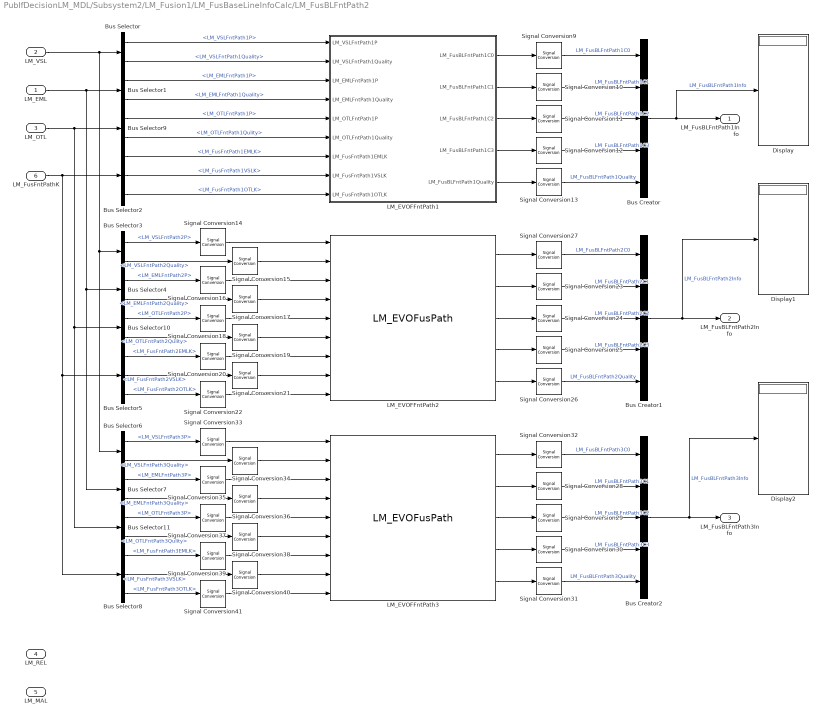
== system PubIfDecisionLM_MDL/Subsystem2/LM_Fusion1/LM_FusBaseLineInfoCalc/LM_FusBLFntPath2 ==
  LM_EML : Inport
  LM_VSL : Inport  Port=2
  LM_OTL : Inport  Port=3
  LM_REL : Inport  Port=4
  LM_MAL : Inport  Port=5
  LM_FusFntPathK : Inport  Port=6
  Bus Creator : BusCreator  Inputs=5
  Bus Creator1 : BusCreator  Inputs=5
  Bus Creator2 : BusCreator  Inputs=5
  Bus Selector : BusSelector  OutputSignals=LM_VSLFntPath1P,LM_VSLFntPath1Quality
  Bus Selector1 : BusSelector  OutputSignals=LM_EMLFntPath1P,LM_EMLFntPath1Quality
  Bus Selector10 : BusSelector  OutputSignals=LM_OTLFntPath2P,LM_OTLFntPath2Qulity
  Bus Selector11 : BusSelector  OutputSignals=LM_OTLFntPath3P,LM_OTLFntPath3Qulity
  Bus Selector2 : BusSelector  OutputSignals=LM_FusFntPath1EMLK,LM_FusFntPath1VSLK,LM_FusFntPath1OTLK
  Bus Selector3 : BusSelector  OutputSignals=LM_VSLFntPath2P,LM_VSLFntPath2Quality
  Bus Selector4 : BusSelector  OutputSignals=LM_EMLFntPath2P,LM_EMLFntPath2Quality
  Bus Selector5 : BusSelector  OutputSignals=LM_FusFntPath2EMLK,LM_FusFntPath2VSLK,LM_FusFntPath2OTLK
  Bus Selector6 : BusSelector  OutputSignals=LM_VSLFntPath3P,LM_VSLFntPath3Quality
  Bus Selector7 : BusSelector  OutputSignals=LM_EMLFntPath3P,LM_EMLFntPath3Quality
  Bus Selector8 : BusSelector  OutputSignals=LM_FusFntPath3EMLK,LM_FusFntPath3VSLK,LM_FusFntPath3OTLK
  Bus Selector9 : BusSelector  OutputSignals=LM_OTLFntPath1P,LM_OTLFntPath1Qulity
  Display : Display
  Display1 : Display
  Display2 : Display
  LM_EVOFFntPath1 : Subsystem
  LM_EVOFFntPath2 : LM_LIB/LM_EVOFusPath  SystemSampleTime=-1  VariantActivationTime=update diagram  Latency=0  AutoFrameSizeCalculation=off
  LM_EVOFFntPath3 : LM_LIB/LM_EVOFusPath  SystemSampleTime=-1  VariantActivationTime=update diagram  Latency=0  AutoFrameSizeCalculation=off
  Signal Conversion{9..41} (33 alike) : SignalConversion  OverrideOpt=off
  LM_FusBLFntPath1Info : Outport
  LM_FusBLFntPath2Info : Outport  Port=2
  LM_FusBLFntPath3Info : Outport  Port=3
  wires:
  Signal Conversion41/1 -> LM_EVOFFntPath3/9
  Signal Conversion40/1 -> LM_EVOFFntPath3/8
  Signal Conversion39/1 -> LM_EVOFFntPath3/7
  Signal Conversion38/1 -> LM_EVOFFntPath3/6
  Signal Conversion37/1 -> LM_EVOFFntPath3/5
  Signal Conversion36/1 -> LM_EVOFFntPath3/4
  Signal Conversion34/1 -> LM_EVOFFntPath3/2
  Signal Conversion35/1 -> LM_EVOFFntPath3/3
  Signal Conversion33/1 -> LM_EVOFFntPath3/1
  Signal Conversion20/1 -> LM_EVOFFntPath2/7
  Signal Conversion18/1 -> LM_EVOFFntPath2/5
  Signal Conversion21/1 -> LM_EVOFFntPath2/8
  Signal Conversion15/1 -> LM_EVOFFntPath2/2
  Signal Conversion19/1 -> LM_EVOFFntPath2/6
  Signal Conversion17/1 -> LM_EVOFFntPath2/4
  Signal Conversion16/1 -> LM_EVOFFntPath2/3
  Signal Conversion14/1 -> LM_EVOFFntPath2/1
  Signal Conversion22/1 -> LM_EVOFFntPath2/9
  Signal Conversion32/1 -> Bus Creator2/1  "LM_FusBLFntPath3C0"
  Signal Conversion31/1 -> Bus Creator2/5  "LM_FusBLFntPath3Quality"
  Signal Conversion30/1 -> Bus Creator2/4  "LM_FusBLFntPath3C3"
  Signal Conversion28/1 -> Bus Creator2/2  "LM_FusBLFntPath3C1"
  Signal Conversion29/1 -> Bus Creator2/3  "LM_FusBLFntPath3C2"
  Signal Conversion23/1 -> Bus Creator1/2  "LM_FusBLFntPath2C1"
  Signal Conversion27/1 -> Bus Creator1/1  "LM_FusBLFntPath2C0"
  Signal Conversion26/1 -> Bus Creator1/5  "LM_FusBLFntPath2Quality"
  Signal Conversion25/1 -> Bus Creator1/4  "LM_FusBLFntPath2C3"
  Signal Conversion24/1 -> Bus Creator1/3  "LM_FusBLFntPath2C2"
  Signal Conversion13/1 -> Bus Creator/5  "LM_FusBLFntPath1Quality"
  Signal Conversion12/1 -> Bus Creator/4  "LM_FusBLFntPath1C3"
  Signal Conversion11/1 -> Bus Creator/3  "LM_FusBLFntPath1C2"
  Signal Conversion10/1 -> Bus Creator/2  "LM_FusBLFntPath1C1"
  Signal Conversion9/1 -> Bus Creator/1  "LM_FusBLFntPath1C0"
  Bus Selector5/2 -> Signal Conversion21/1  "<LM_FusFntPath2VSLK>"
  Bus Selector2/1 -> LM_EVOFFntPath1/7(LM_FusFntPath1EMLK)  "<LM_FusFntPath1EMLK>"
  LM_EVOFFntPath3/5 -> Signal Conversion31/1
  LM_EVOFFntPath3/4 -> Signal Conversion30/1
  LM_EVOFFntPath3/3 -> Signal Conversion29/1
  LM_EVOFFntPath3/2 -> Signal Conversion28/1
  LM_EVOFFntPath3/1 -> Signal Conversion32/1
  Bus Selector8/3 -> Signal Conversion41/1  "<LM_FusFntPath3OTLK>"
  Bus Selector11/2 -> Signal Conversion38/1  "<LM_OTLFntPath3Qulity>"
  Bus Selector11/1 -> Signal Conversion37/1  "<LM_OTLFntPath3P>"
  LM_EVOFFntPath2/5 -> Signal Conversion26/1
  LM_EVOFFntPath2/4 -> Signal Conversion25/1
  LM_EVOFFntPath2/3 -> Signal Conversion24/1
  LM_EVOFFntPath2/2 -> Signal Conversion23/1
  LM_EVOFFntPath2/1 -> Signal Conversion27/1
  Bus Selector5/3 -> Signal Conversion22/1  "<LM_FusFntPath2OTLK>"
  Bus Selector10/2 -> Signal Conversion19/1  "<LM_OTLFntPath2Qulity>"
  Bus Selector10/1 -> Signal Conversion18/1  "<LM_OTLFntPath2P>"
  Bus Selector2/3 -> LM_EVOFFntPath1/9(LM_FusFntPath1OTLK)  "<LM_FusFntPath1OTLK>"
  LM_OTL/1 -> Bus Selector9/1, Bus Selector10/1, Bus Selector11/1
  Bus Selector9/2 -> LM_EVOFFntPath1/6(LM_OTLFntPath1Quality)  "<LM_OTLFntPath1Qulity>"
  Bus Selector9/1 -> LM_EVOFFntPath1/5(LM_OTLFntPath1P)  "<LM_OTLFntPath1P>"
  LM_EVOFFntPath1/5(LM_FusBLFntPath1Quality) -> Signal Conversion13/1
  LM_EVOFFntPath1/4(LM_FusBLFntPath1C3) -> Signal Conversion12/1
  LM_EVOFFntPath1/3(LM_FusBLFntPath1C2) -> Signal Conversion11/1
  LM_EVOFFntPath1/2(LM_FusBLFntPath1C1) -> Signal Conversion10/1
  LM_EVOFFntPath1/1(LM_FusBLFntPath1C0) -> Signal Conversion9/1
  Bus Selector8/2 -> Signal Conversion40/1  "<LM_FusFntPath3VSLK>"
  Bus Selector8/1 -> Signal Conversion39/1  "<LM_FusFntPath3EMLK>"
  Bus Selector7/2 -> Signal Conversion36/1  "<LM_EMLFntPath3Quality>"
  Bus Selector7/1 -> Signal Conversion35/1  "<LM_EMLFntPath3P>"
  Bus Selector6/2 -> Signal Conversion34/1  "<LM_VSLFntPath3Quality>"
  Bus Selector6/1 -> Signal Conversion33/1  "<LM_VSLFntPath3P>"
  Bus Selector5/1 -> Signal Conversion20/1  "<LM_FusFntPath2EMLK>"
  Bus Selector4/2 -> Signal Conversion17/1  "<LM_EMLFntPath2Quality>"
  Bus Selector4/1 -> Signal Conversion16/1  "<LM_EMLFntPath2P>"
  Bus Selector3/2 -> Signal Conversion15/1  "<LM_VSLFntPath2Quality>"
  Bus Selector3/1 -> Signal Conversion14/1  "<LM_VSLFntPath2P>"
  Bus Selector1/2 -> LM_EVOFFntPath1/4(LM_EMLFntPath1Quality)  "<LM_EMLFntPath1Quality>"
  Bus Selector/2 -> LM_EVOFFntPath1/2(LM_VSLFntPath1Quality)  "<LM_VSLFntPath1Quality>"
  LM_FusFntPathK/1 -> Bus Selector8/1, Bus Selector5/1, Bus Selector2/1
  LM_VSL/1 -> Bus Selector/1, Bus Selector3/1, Bus Selector6/1
  LM_EML/1 -> Bus Selector1/1, Bus Selector4/1, Bus Selector7/1
  Bus Creator/1 -> LM_FusBLFntPath1Info/1, Display/1  "LM_FusBLFntPath1Info"
  Bus Creator1/1 -> LM_FusBLFntPath2Info/1, Display1/1  "LM_FusBLFntPath2Info"
  Bus Selector1/1 -> LM_EVOFFntPath1/3(LM_EMLFntPath1P)  "<LM_EMLFntPath1P>"
  Bus Creator2/1 -> LM_FusBLFntPath3Info/1, Display2/1  "LM_FusBLFntPath3Info"
  Bus Selector/1 -> LM_EVOFFntPath1/1(LM_VSLFntPath1P)  "<LM_VSLFntPath1P>"
  Bus Selector2/2 -> LM_EVOFFntPath1/8(LM_FusFntPath1VSLK)  "<LM_FusFntPath1VSLK>"

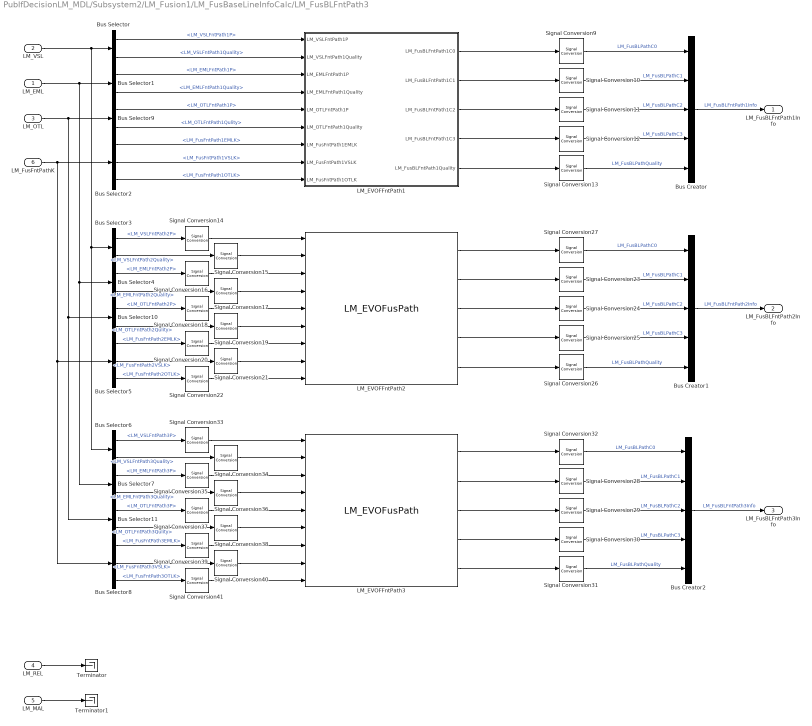
== system PubIfDecisionLM_MDL/Subsystem2/LM_Fusion1/LM_FusBaseLineInfoCalc/LM_FusBLFntPath3 ==
  LM_EML : Inport
  LM_VSL : Inport  Port=2
  LM_OTL : Inport  Port=3
  LM_REL : Inport  Port=4
  LM_MAL : Inport  Port=5
  LM_FusFntPathK : Inport  Port=6
  Bus Creator : BusCreator  Inputs=5  OutDataTypeStr=Bus: LM_FusBLPathInfoBus
  Bus Creator1 : BusCreator  Inputs=5  OutDataTypeStr=Bus: LM_FusBLPathInfoBus
  Bus Creator2 : BusCreator  Inputs=5  OutDataTypeStr=Bus: LM_FusBLPathInfoBus
  Bus Selector : BusSelector  OutputSignals=LM_VSLFntPath1P,LM_VSLFntPath1Quality
  Bus Selector1 : BusSelector  OutputSignals=LM_EMLFntPath1P,LM_EMLFntPath1Quality
  Bus Selector10 : BusSelector  OutputSignals=LM_OTLFntPath2P,LM_OTLFntPath2Qulity
  Bus Selector11 : BusSelector  OutputSignals=LM_OTLFntPath3P,LM_OTLFntPath3Qulity
  Bus Selector2 : BusSelector  OutputSignals=LM_FusFntPath1EMLK,LM_FusFntPath1VSLK,LM_FusFntPath1OTLK
  Bus Selector3 : BusSelector  OutputSignals=LM_VSLFntPath2P,LM_VSLFntPath2Quality
  Bus Selector4 : BusSelector  OutputSignals=LM_EMLFntPath2P,LM_EMLFntPath2Quality
  Bus Selector5 : BusSelector  OutputSignals=LM_FusFntPath2EMLK,LM_FusFntPath2VSLK,LM_FusFntPath2OTLK
  Bus Selector6 : BusSelector  OutputSignals=LM_VSLFntPath3P,LM_VSLFntPath3Quality
  Bus Selector7 : BusSelector  OutputSignals=LM_EMLFntPath3P,LM_EMLFntPath3Quality
  Bus Selector8 : BusSelector  OutputSignals=LM_FusFntPath3EMLK,LM_FusFntPath3VSLK,LM_FusFntPath3OTLK
  Bus Selector9 : BusSelector  OutputSignals=LM_OTLFntPath1P,LM_OTLFntPath1Qulity
  LM_EVOFFntPath1 : Subsystem
  LM_EVOFFntPath2 : LM_LIB/LM_EVOFusPath  SystemSampleTime=-1  VariantActivationTime=update diagram  Latency=0  AutoFrameSizeCalculation=off
  LM_EVOFFntPath3 : LM_LIB/LM_EVOFusPath  SystemSampleTime=-1  VariantActivationTime=update diagram  Latency=0  AutoFrameSizeCalculation=off
  Signal Conversion{9..41} (33 alike) : SignalConversion  OverrideOpt=off
  Terminator : Terminator
  Terminator1 : Terminator
  LM_FusBLFntPath1Info : Outport
  LM_FusBLFntPath2Info : Outport  Port=2
  LM_FusBLFntPath3Info : Outport  Port=3
  wires:
  Bus Selector2/2 -> LM_EVOFFntPath1/8(LM_FusFntPath1VSLK)  "<LM_FusFntPath1VSLK>"
  Bus Selector/1 -> LM_EVOFFntPath1/1(LM_VSLFntPath1P)  "<LM_VSLFntPath1P>"
  Bus Selector1/1 -> LM_EVOFFntPath1/3(LM_EMLFntPath1P)  "<LM_EMLFntPath1P>"
  LM_EML/1 -> Bus Selector7/1, Bus Selector4/1, Bus Selector1/1
  LM_VSL/1 -> Bus Selector6/1, Bus Selector3/1, Bus Selector/1
  LM_FusFntPathK/1 -> Bus Selector2/1, Bus Selector8/1, Bus Selector5/1
  Bus Selector/2 -> LM_EVOFFntPath1/2(LM_VSLFntPath1Quality)  "<LM_VSLFntPath1Quality>"
  Bus Selector1/2 -> LM_EVOFFntPath1/4(LM_EMLFntPath1Quality)  "<LM_EMLFntPath1Quality>"
  Bus Selector3/1 -> Signal Conversion14/1  "<LM_VSLFntPath2P>"
  Bus Selector3/2 -> Signal Conversion15/1  "<LM_VSLFntPath2Quality>"
  Bus Selector4/1 -> Signal Conversion16/1  "<LM_EMLFntPath2P>"
  Bus Selector4/2 -> Signal Conversion17/1  "<LM_EMLFntPath2Quality>"
  Bus Selector5/1 -> Signal Conversion20/1  "<LM_FusFntPath2EMLK>"
  Bus Selector6/1 -> Signal Conversion33/1  "<LM_VSLFntPath3P>"
  Bus Selector6/2 -> Signal Conversion34/1  "<LM_VSLFntPath3Quality>"
  Bus Selector7/1 -> Signal Conversion35/1  "<LM_EMLFntPath3P>"
  Bus Selector7/2 -> Signal Conversion36/1  "<LM_EMLFntPath3Quality>"
  Bus Selector8/1 -> Signal Conversion39/1  "<LM_FusFntPath3EMLK>"
  Bus Selector8/2 -> Signal Conversion40/1  "<LM_FusFntPath3VSLK>"
  LM_EVOFFntPath1/1(LM_FusBLFntPath1C0) -> Signal Conversion9/1
  LM_EVOFFntPath1/2(LM_FusBLFntPath1C1) -> Signal Conversion10/1
  LM_EVOFFntPath1/3(LM_FusBLFntPath1C2) -> Signal Conversion11/1
  LM_EVOFFntPath1/4(LM_FusBLFntPath1C3) -> Signal Conversion12/1
  LM_EVOFFntPath1/5(LM_FusBLFntPath1Quality) -> Signal Conversion13/1
  Bus Selector9/1 -> LM_EVOFFntPath1/5(LM_OTLFntPath1P)  "<LM_OTLFntPath1P>"
  Bus Selector9/2 -> LM_EVOFFntPath1/6(LM_OTLFntPath1Quality)  "<LM_OTLFntPath1Qulity>"
  LM_OTL/1 -> Bus Selector11/1, Bus Selector10/1, Bus Selector9/1
  Bus Selector2/3 -> LM_EVOFFntPath1/9(LM_FusFntPath1OTLK)  "<LM_FusFntPath1OTLK>"
  Bus Selector10/1 -> Signal Conversion18/1  "<LM_OTLFntPath2P>"
  Bus Selector10/2 -> Signal Conversion19/1  "<LM_OTLFntPath2Qulity>"
  Bus Selector5/3 -> Signal Conversion22/1  "<LM_FusFntPath2OTLK>"
  LM_EVOFFntPath2/1 -> Signal Conversion27/1
  LM_EVOFFntPath2/2 -> Signal Conversion23/1
  LM_EVOFFntPath2/3 -> Signal Conversion24/1
  LM_EVOFFntPath2/4 -> Signal Conversion25/1
  LM_EVOFFntPath2/5 -> Signal Conversion26/1
  Bus Selector11/1 -> Signal Conversion37/1  "<LM_OTLFntPath3P>"
  Bus Selector11/2 -> Signal Conversion38/1  "<LM_OTLFntPath3Qulity>"
  Bus Selector8/3 -> Signal Conversion41/1  "<LM_FusFntPath3OTLK>"
  LM_EVOFFntPath3/1 -> Signal Conversion32/1
  LM_EVOFFntPath3/2 -> Signal Conversion28/1
  LM_EVOFFntPath3/3 -> Signal Conversion29/1
  LM_EVOFFntPath3/4 -> Signal Conversion30/1
  LM_EVOFFntPath3/5 -> Signal Conversion31/1
  Bus Selector2/1 -> LM_EVOFFntPath1/7(LM_FusFntPath1EMLK)  "<LM_FusFntPath1EMLK>"
  Bus Selector5/2 -> Signal Conversion21/1  "<LM_FusFntPath2VSLK>"
  Signal Conversion9/1 -> Bus Creator/1  "LM_FusBLPathC0"
  Signal Conversion10/1 -> Bus Creator/2  "LM_FusBLPathC1"
  Signal Conversion11/1 -> Bus Creator/3  "LM_FusBLPathC2"
  Signal Conversion12/1 -> Bus Creator/4  "LM_FusBLPathC3"
  Signal Conversion13/1 -> Bus Creator/5  "LM_FusBLPathQuality"
  Signal Conversion22/1 -> LM_EVOFFntPath2/9
  Signal Conversion14/1 -> LM_EVOFFntPath2/1
  Signal Conversion16/1 -> LM_EVOFFntPath2/3
  Signal Conversion17/1 -> LM_EVOFFntPath2/4
  Signal Conversion19/1 -> LM_EVOFFntPath2/6
  Signal Conversion15/1 -> LM_EVOFFntPath2/2
  Signal Conversion21/1 -> LM_EVOFFntPath2/8
  Signal Conversion18/1 -> LM_EVOFFntPath2/5
  Signal Conversion20/1 -> LM_EVOFFntPath2/7
  Signal Conversion33/1 -> LM_EVOFFntPath3/1
  Signal Conversion35/1 -> LM_EVOFFntPath3/3
  Signal Conversion34/1 -> LM_EVOFFntPath3/2
  Signal Conversion36/1 -> LM_EVOFFntPath3/4
  Signal Conversion37/1 -> LM_EVOFFntPath3/5
  Signal Conversion38/1 -> LM_EVOFFntPath3/6
  Signal Conversion39/1 -> LM_EVOFFntPath3/7
  Signal Conversion40/1 -> LM_EVOFFntPath3/8
  Signal Conversion41/1 -> LM_EVOFFntPath3/9
  LM_REL/1 -> Terminator/1
  LM_MAL/1 -> Terminator1/1
  Bus Creator/1 -> LM_FusBLFntPath1Info/1  "LM_FusBLFntPath1Info"
  Bus Creator1/1 -> LM_FusBLFntPath2Info/1  "LM_FusBLFntPath2Info"
  Bus Creator2/1 -> LM_FusBLFntPath3Info/1  "LM_FusBLFntPath3Info"
  Signal Conversion26/1 -> Bus Creator1/5  "LM_FusBLPathQuality"
  Signal Conversion25/1 -> Bus Creator1/4  "LM_FusBLPathC3"
  Signal Conversion24/1 -> Bus Creator1/3  "LM_FusBLPathC2"
  Signal Conversion23/1 -> Bus Creator1/2  "LM_FusBLPathC1"
  Signal Conversion27/1 -> Bus Creator1/1  "LM_FusBLPathC0"
  Signal Conversion32/1 -> Bus Creator2/1  "LM_FusBLPathC0"
  Signal Conversion28/1 -> Bus Creator2/2  "LM_FusBLPathC1"
  Signal Conversion29/1 -> Bus Creator2/3  "LM_FusBLPathC2"
  Signal Conversion30/1 -> Bus Creator2/4  "LM_FusBLPathC3"
  Signal Conversion31/1 -> Bus Creator2/5  "LM_FusBLPathQuality"
